simulink subsystem "DCMotor"  (R2020a)
settings: Solver=VariableStepAuto  StartTime=0.0  StopTime=10.0  RelTol=1e-3
settings Model: Creator=Thomas  LastModifiedBy=Thomas

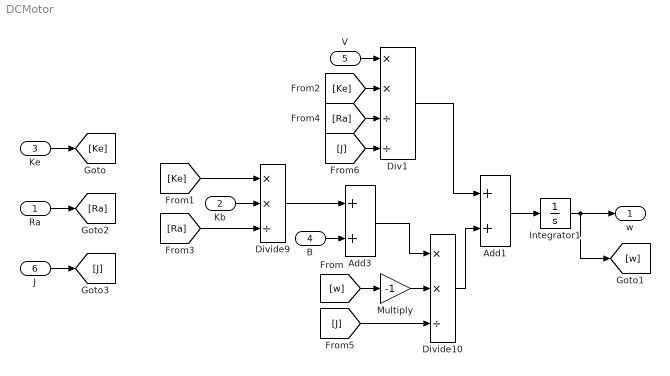
== system DCMotor ==
  Ra : Inport
  Kb : Inport  Port=2
  Ke : Inport  Port=3
  B : Inport  Port=4
  V : Inport  Port=5
  J : Inport  Port=6
  Add1 : Sum
  Add3 : Sum
  Div1 : Product  Inputs=**//
  Divide10 : Product  Inputs=**/
  Divide9 : Product  Inputs=**/
  Integrator1 : Integrator
  Multiply : Gain  Gain=-1
  w : Outport
  wires:
  Ke/1 -> [Ke]
  [w] -> Multiply/1
  Kb/1 -> Divide9/2
  Add3/1 -> Divide10/1
  Divide9/1 -> Add3/1
  Integrator1/1 -> w/1, [w]
  B/1 -> Add3/2
  Multiply/1 -> Divide10/2
  V/1 -> Div1/1
  Divide10/1 -> Add1/2
  Div1/1 -> Add1/1
  Add1/1 -> Integrator1/1
  [Ke] -> Divide9/1
  [Ke] -> Div1/2
  Ra/1 -> [Ra]
  [Ra] -> Divide9/3
  [Ra] -> Div1/3
  J/1 -> [J]
  [J] -> Divide10/3
  [J] -> Div1/4
